simulink model "APV_RL_breach"  (R2021a)
settings: Solver=FixedStepAuto  StartTime=0.0  StopTime=T  FixedStep=Ts  RelTol=1e-3
undefined symbols (not defined in the file): info, max_theta_error, max_x_error, max_y_error, pTracking, theta_error_offset, Ts, x_error_offset, y_error_offset
libraries: simulink x3, robotmobilelib x1, simulink_extras x1, mpclib x1, rllib x1
settings Model: Creator=The MathWorks, Inc.  LastModifiedBy=ldy
settings SolverCC: AlgebraicLoopSolver=TrustRegion
settings DebuggingCC: SFMachineParentedDataDiag=warning

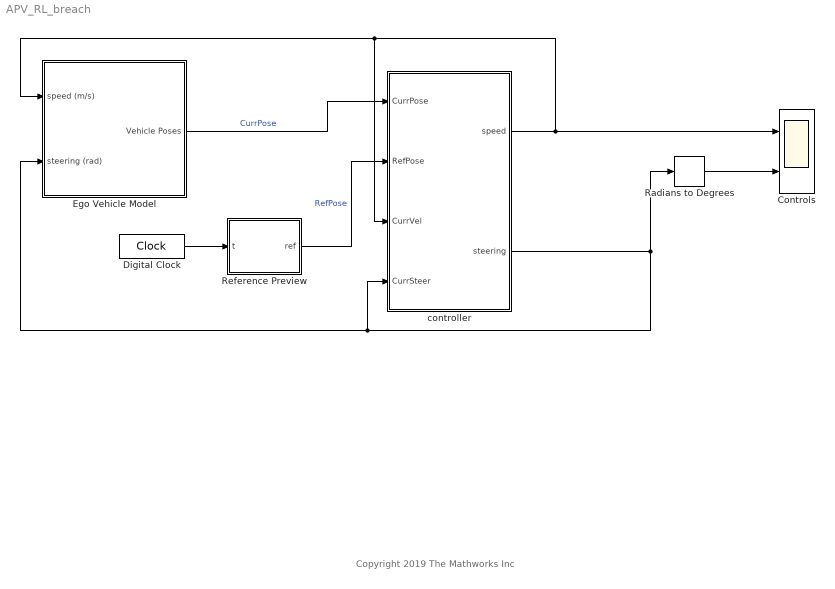
== system APV_RL_breach ==
  note: Copyright 2019 The Mathworks Inc
  Controls : Scope  NumInputPorts=2
  Digital Clock : DigitalClock  SampleTime=Ts
  Ego Vehicle Model : Subsystem
  Radians to Degrees : simulink_extras/Transformations/Radians to Degrees
  Reference Preview : MATLAB Function  TreatAsAtomicUnit=on
  controller : Subsystem
  wires:
  Radians to Degrees/1 -> Controls/2
  Digital Clock/1 -> Reference Preview/1(t)
  controller/1(speed) -> Controls/1, controller/3(CurrVel), Ego Vehicle Model/1(speed (m/s))
  controller/2(steering) -> Radians to Degrees/1, controller/4(CurrSteer), Ego Vehicle Model/2(steering (rad))
  Ego Vehicle Model/1(Vehicle Poses) -> controller/1(CurrPose)  "CurrPose"
  Reference Preview/1(ref) -> controller/2(RefPose)  "RefPose"

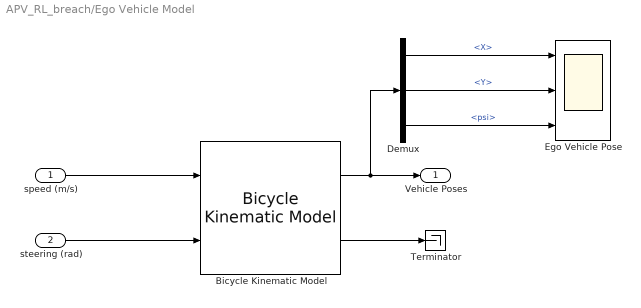
== system APV_RL_breach/Ego Vehicle Model ==
  speed (m/s) : Inport
  steering (rad) : Inport  Port=2
  Bicycle Kinematic Model : robotmobilelib/Bicycle Kinematic Model  VehicleInputs=Vehicle Speed & Steering Angle  WheelBase=2.8  VehicleSpeedRange=[-6.5 6.5]  MaxSteeringAngle=pi/4  InitialState=egoInitialPose  SimulateUsing=Interpreted execution
      settings: SourceProductBaseCode=RO
  Demux : Demux  Outputs=3
  Ego Vehicle Pose : Scope  NumInputPorts=3
  Terminator : Terminator
  Vehicle Poses : Outport
  wires:
  Bicycle Kinematic Model/1 -> Demux/1, Vehicle Poses/1
  speed (m/s)/1 -> Bicycle Kinematic Model/1
  steering (rad)/1 -> Bicycle Kinematic Model/2
  Bicycle Kinematic Model/2 -> Terminator/1
  Demux/3 -> Ego Vehicle Pose/3  "<psi>"
  Demux/2 -> Ego Vehicle Pose/2  "<Y>"
  Demux/1 -> Ego Vehicle Pose/1  "<X>"

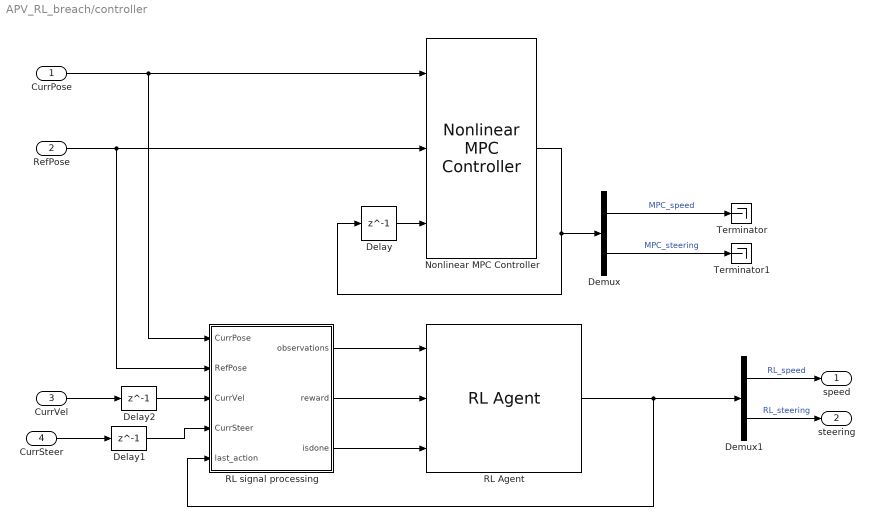
== system APV_RL_breach/controller ==
  CurrPose : Inport
  RefPose : Inport  Port=2
  CurrVel : Inport  Port=3
  CurrSteer : Inport  Port=4
  Delay : Delay  DelayLength=1
  Delay1 : Delay  DelayLength=1
  Delay2 : Delay  DelayLength=1
  Demux : Demux  Outputs=[1 1]
  Demux1 : Demux  Outputs=[1 1]
  Nonlinear MPC Controller : mpclib/Nonlinear MPC Controller  SCDEnableBlockLinearizationSpecification=on  nlmpcobj=nlobjTracking  UseObjectTs=on  UseMEX=off  mexname=''  md_enabled=off  mvtarget_enabled=off  param_enabled=off  cost_enabled=off  mvseq_enabled=off  stateseq_enabled=off  ovseq_enabled=off  slack_enabled=off  status_enabled=off  ov_min=off  ov_max=off  mv_min=off  mv_max=off  mvrate_min=off  mvrate_max=off  state_min=off  state_max=off  ov_weight=off  mv_weight=off  mvrate_weight=off  ecr_weight=off  nlp_initialize=off
  RL Agent : rllib/RL Agent  Agent=agent  ExternalActionAsInput=off  ProvideCumRwd=off  TreatAsDirectFeedthrough=on
  RL signal processing : Subsystem
  Terminator : Terminator
  Terminator1 : Terminator
  speed : Outport
  steering : Outport  Port=2
  wires:
  CurrPose/1 -> RL signal processing/1(CurrPose), Nonlinear MPC Controller/1
  Nonlinear MPC Controller/1 -> Delay/1, Demux/1
  Delay/1 -> Nonlinear MPC Controller/3
  RefPose/1 -> RL signal processing/2(RefPose), Nonlinear MPC Controller/2
  Demux/1 -> Terminator/1  "MPC_speed"
  Demux/2 -> Terminator1/1  "MPC_steering"
  RL signal processing/1(observations) -> RL Agent/1
  RL signal processing/2(reward) -> RL Agent/2
  RL signal processing/3(isdone) -> RL Agent/3
  Demux1/1 -> speed/1  "RL_speed"
  Demux1/2 -> steering/1  "RL_steering"
  CurrVel/1 -> Delay2/1
  CurrSteer/1 -> Delay1/1
  Delay2/1 -> RL signal processing/3(CurrVel)
  Delay1/1 -> RL signal processing/4(CurrSteer)
  RL Agent/1 -> RL signal processing/5(last_action), Demux1/1

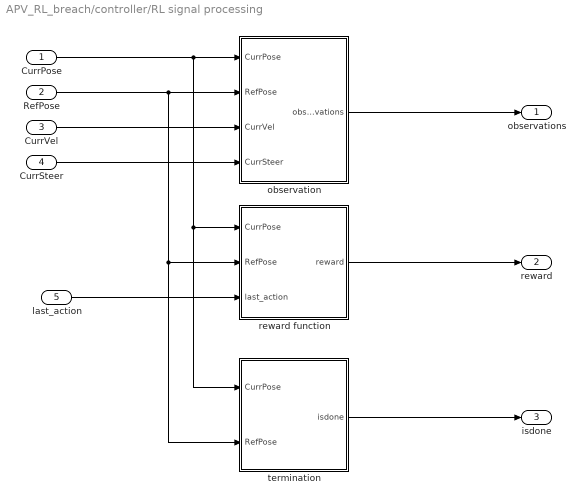
== system APV_RL_breach/controller/RL signal processing ==
  CurrPose : Inport
  RefPose : Inport  Port=2
  CurrVel : Inport  Port=3
  CurrSteer : Inport  Port=4
  last_action : Inport  Port=5
  observation : Subsystem
  reward function : Subsystem
  termination : Subsystem
  observations : Outport
  reward : Outport  Port=2
  isdone : Outport  Port=3
  wires:
  CurrPose/1 -> termination/1(CurrPose), reward function/1(CurrPose), observation/1(CurrPose)
  observation/1(observations) -> observations/1
  RefPose/1 -> termination/2(RefPose), reward function/2(RefPose), observation/2(RefPose)
  termination/1(isdone) -> isdone/1
  reward function/1(reward) -> reward/1
  CurrVel/1 -> observation/3(CurrVel)
  CurrSteer/1 -> observation/4(CurrSteer)
  last_action/1 -> reward function/3(last_action)

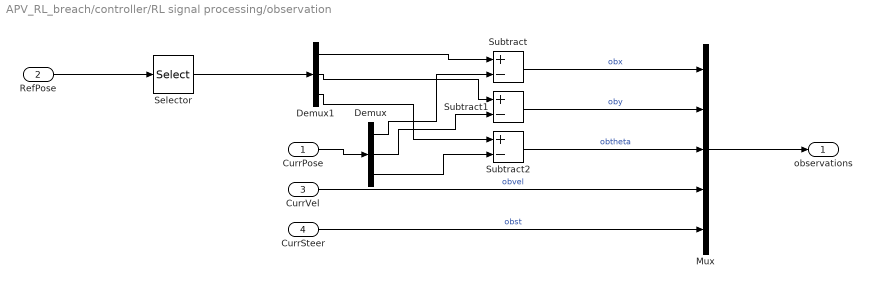
== system APV_RL_breach/controller/RL signal processing/observation ==
  CurrPose : Inport
  RefPose : Inport  Port=2
  CurrVel : Inport  Port=3
  CurrSteer : Inport  Port=4
  Demux : Demux  Outputs=3
  Demux1 : Demux  Outputs=3
  Mux : Mux  Inputs=5
  Selector : Selector  NumberOfDimensions=2  InputPortWidth=3  IndexOptions=Index vector (dialog),Index vector (dialog)  Indices=1,[1:3]  OutputSizes=1,1
  Subtract : Sum  Inputs=+-
  Subtract1 : Sum  Inputs=+-
  Subtract2 : Sum  Inputs=+-
  observations : Outport
  wires:
  CurrPose/1 -> Demux/1
  RefPose/1 -> Selector/1
  Selector/1 -> Demux1/1
  CurrSteer/1 -> Mux/5  "obst"
  CurrVel/1 -> Mux/4  "obvel"
  Demux/1 -> Subtract/2
  Subtract/1 -> Mux/1  "obx"
  Demux/2 -> Subtract1/2
  Demux/3 -> Subtract2/2
  Subtract2/1 -> Mux/3  "obtheta"
  Subtract1/1 -> Mux/2  "oby"
  Demux1/1 -> Subtract/1
  Demux1/2 -> Subtract1/1
  Demux1/3 -> Subtract2/1
  Mux/1 -> observations/1

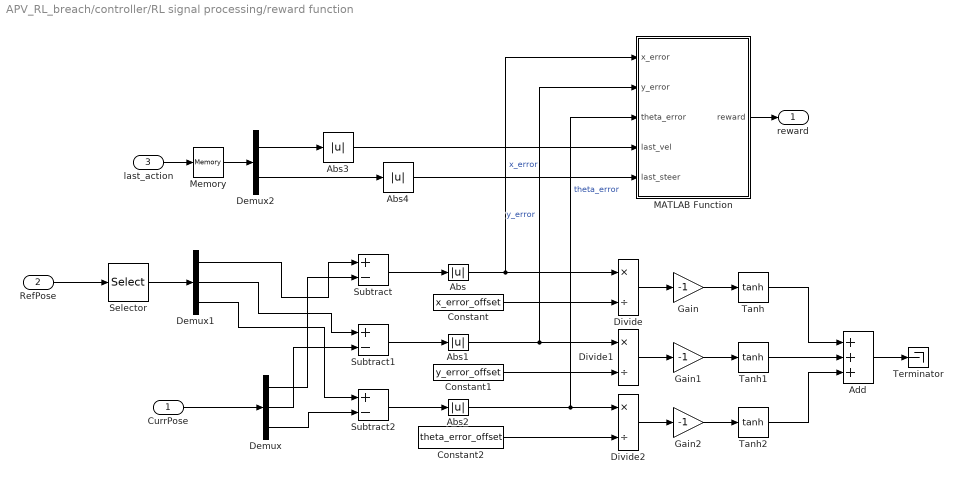
== system APV_RL_breach/controller/RL signal processing/reward function ==
  CurrPose : Inport
  RefPose : Inport  Port=2
  last_action : Inport  Port=3
  Abs{,1..4} (5 alike) : Abs
  Add : Sum  Inputs=+++
  Constant : Constant  Value=x_error_offset
  Constant1 : Constant  Value=y_error_offset
  Constant2 : Constant  Value=theta_error_offset
  Demux : Demux  Outputs=3
  Demux1 : Demux  Outputs=3
  Demux2 : Demux  Outputs=[1 1]
  Divide : Product  Inputs=*/
  Divide1 : Product  Inputs=*/
  Divide2 : Product  Inputs=*/
  Gain : Gain  Gain=-1
  Gain1 : Gain  Gain=-1
  Gain2 : Gain  Gain=-1
  MATLAB Function : MATLAB Function  TreatAsAtomicUnit=on
  Memory : Memory
  Selector : Selector  NumberOfDimensions=2  InputPortWidth=3  IndexOptions=Index vector (dialog),Index vector (dialog)  Indices=1,[1:3]  OutputSizes=1,1
  Subtract : Sum  Inputs=+-
  Subtract1 : Sum  Inputs=+-
  Subtract2 : Sum  Inputs=+-
  Tanh : Trigonometry  Operator=tanh
  Tanh1 : Trigonometry  Operator=tanh
  Tanh2 : Trigonometry  Operator=tanh
  Terminator : Terminator
  reward : Outport
  wires:
  Selector/1 -> Demux1/1
  Demux/3 -> Subtract2/2
  Demux/2 -> Subtract1/2
  CurrPose/1 -> Demux/1
  Demux/1 -> Subtract/2
  RefPose/1 -> Selector/1
  Abs2/1 -> MATLAB Function/3(theta_error), Divide2/1  "theta_error"
  Abs1/1 -> MATLAB Function/2(y_error), Divide1/1  "y_error"
  Abs/1 -> MATLAB Function/1(x_error), Divide/1  "x_error"
  Tanh/1 -> Add/1
  Gain1/1 -> Tanh1/1
  Divide/1 -> Gain/1
  Gain/1 -> Tanh/1
  Tanh1/1 -> Add/2
  Constant/1 -> Divide/2
  Divide1/1 -> Gain1/1
  Divide2/1 -> Gain2/1
  Gain2/1 -> Tanh2/1
  Tanh2/1 -> Add/3
  Constant2/1 -> Divide2/2
  Constant1/1 -> Divide1/2
  Subtract/1 -> Abs/1
  Subtract1/1 -> Abs1/1
  Subtract2/1 -> Abs2/1
  Demux1/1 -> Subtract/1
  Demux1/2 -> Subtract1/1
  Demux1/3 -> Subtract2/1
  MATLAB Function/1(reward) -> reward/1
  Add/1 -> Terminator/1
  last_action/1 -> Memory/1
  Memory/1 -> Demux2/1
  Demux2/1 -> Abs3/1
  Demux2/2 -> Abs4/1
  Abs3/1 -> MATLAB Function/4(last_vel)
  Abs4/1 -> MATLAB Function/5(last_steer)

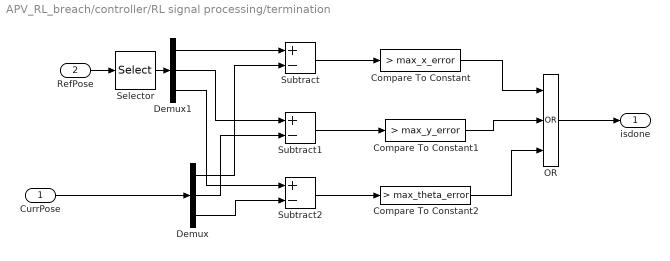
== system APV_RL_breach/controller/RL signal processing/termination ==
  CurrPose : Inport
  RefPose : Inport  Port=2
  Compare To Constant : simulink/Logic and Bit Operations/Compare To Constant  relop=>  const=max_x_error  OutDataTypeStr=boolean
  Compare To Constant1 : simulink/Logic and Bit Operations/Compare To Constant  relop=>  const=max_y_error  OutDataTypeStr=boolean
  Compare To Constant2 : simulink/Logic and Bit Operations/Compare To Constant  relop=>  const=max_theta_error  OutDataTypeStr=boolean
  Demux : Demux  Outputs=3
  Demux1 : Demux  Outputs=3
  OR : Logic  Operator=OR  Inputs=3  IconShape=distinctive  AllPortsSameDT=off  OutDataTypeStr=boolean
  Selector : Selector  NumberOfDimensions=2  InputPortWidth=3  IndexOptions=Index vector (dialog),Index vector (dialog)  Indices=1,[1:3]  OutputSizes=1,1
  Subtract : Sum  Inputs=+-
  Subtract1 : Sum  Inputs=+-
  Subtract2 : Sum  Inputs=+-
  isdone : Outport
  wires:
  CurrPose/1 -> Demux/1
  Selector/1 -> Demux1/1
  Demux/2 -> Subtract1/2
  Demux/1 -> Subtract/2
  Demux/3 -> Subtract2/2
  RefPose/1 -> Selector/1
  Subtract/1 -> Compare To Constant/1
  Subtract2/1 -> Compare To Constant2/1
  Subtract1/1 -> Compare To Constant1/1
  Compare To Constant/1 -> OR/1
  Compare To Constant1/1 -> OR/2
  Compare To Constant2/1 -> OR/3
  OR/1 -> isdone/1
  Demux1/1 -> Subtract/1
  Demux1/2 -> Subtract1/1
  Demux1/3 -> Subtract2/1

== matlab function APV_RL_breach/Reference Preview ==
  data: t input; ref output; Ts parameter; info parameter; pTracking parameter
function ref = fcn(t,Ts,info,pTracking)
Tend = info.Topt(end);
T = t+(1:pTracking)*Ts;
T = min(T,Tend);
ref = interp1(info.Topt,info.Xopt(:,1:3),T);

== matlab function APV_RL_breach/controller/RL signal processing/reward function/MATLAB Function ==
  data: x_error input; reward output; y_error input; theta_error input; last_vel input; last_steer input
function reward = reward(x_error, y_error, theta_error, last_vel, last_steer)

x_pos = 2*exp(-x_error*1.5);
y_pos = 2*exp(-y_error*1.5);
theta_pos = 2*exp(-theta_error*1.5);

neg_reward = -tanh(x_error) -tanh(y_pos) -tanh(theta_pos) ;

reward = x_pos + y_pos + theta_pos + neg_reward - 0.01*last_vel - 0.1*last_steer;
